simulink model "Improved_EKFSim"  (R2021b)
settings: Solver=VariableStepAuto  StartTime=0.0  StopTime=12000  RelTol=1e-3
undefined symbols (not defined in the file): sigbuilder_block
libraries: commchan3 x2
settings Model: Creator=Lenovo  LastModifiedBy=matthewathanasopoulos
settings SolverCC: AlgebraicLoopSolver=TrustRegion
settings DataIOCC: ReturnWorkspaceOutputs=off
settings DebuggingCC: SFMachineParentedDataDiag=warning  ArithmeticOperatorsInVariantConditions=warning
settings SFSimCC: SimUseLocalCustomCode=off  CustomCodeUndefinedFunction=UseInterfaceOnly
settings RTWCC: RTWUseLocalCustomCode=off

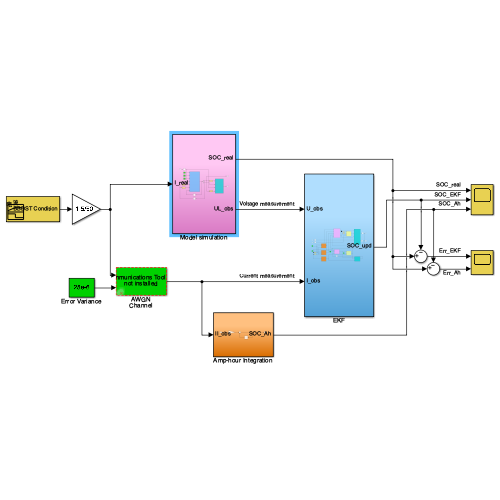
[thumbnail: Simulink's stored preview of the top-level diagram]
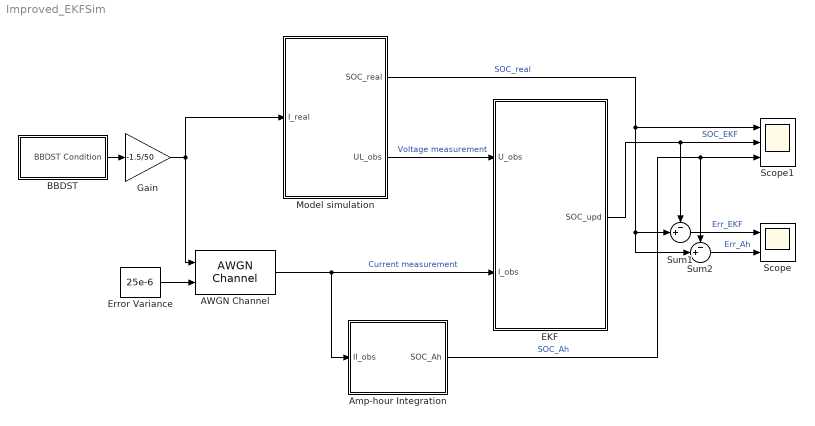
== system Improved_EKFSim ==
  AWGN Channel : commchan3/AWGN Channel  InputProcessing=Columns as channels (frame based)  seed=1  noiseMode=Variance from port  EbNodB=10  EsNodB=10  SNRdB=10  bitsPerSym=1  Ps=1  Tsym=1  variance=1
  Amp-hour Integration : Subsystem
  BBDST : Subsystem  Tag=STV Subsys  LoadFcn=sigbuilder_block('load');  StartFcn=sigbuilder_block('start');  StopFcn=sigbuilder_block('stop');  ClipboardFcn=sigbuilder_block('clipboard');  mask(Sigbuilder block){tuvar=[0:10]}
      mask help: Simulink:masks:SigbuilderBlock_MD
      mask init:
      | if ~strcmp(get_param(bdroot(gcbh),'SimulationStatus'),'stopped') tuvar = sigbuilder_block('maskInit'); end
      settings: CopyFcn=sigbuilder_block('copy');  DeleteFcn=sigbuilder_block('delete');  ModelCloseFcn=sigbuilder_block('modelClose');  PreSaveFcn=sigbuilder_block('preSave');  PauseFcn=sigbuilder_block('pause');  ContinueFcn=sigbuilder_block('continue');  NameChangeFcn=sigbuilder_block('namechange');  OpenFcn=sigbuilder_block('open',[162 96 990 471 ]);  CloseFcn=sigbuilder_block('close');
      mask Display: plot(0, 0, 100, 100,[2, 2, 32, 32, 2], [68, 8, 8, 68, 68],[32, 2], [38, 38], [32, 19, 2],[53, 60, 44], [32, 17, 17, 2],[16, 16, 31, 31]);txt = getActiveGroup(gcbh);text(2, 100, txt,'verticalAlignment', 'top');
  EKF : Subsystem
  Error Variance : Constant  Value=25e-6
  Gain : Gain  Gain=-1.5/50
  Model simulation : Subsystem
  Scope : Scope  NumInputPorts=2
  Scope1 : Scope  NumInputPorts=3
  Sum1 : Sum  Inputs=-+|
  Sum2 : Sum  Inputs=-+|
  wires:
  BBDST/1(BBDST Condition) -> Gain/1
  AWGN Channel/1 -> Amp-hour Integration/1(II_obs), EKF/2(I_obs)  "Current measurement"
  EKF/1(SOC_upd) -> Sum1/1, Scope1/2  "SOC_EKF"
  Model simulation/2(UL_obs) -> EKF/1(U_obs)  "Voltage measurement"
  Model simulation/1(SOC_real) -> Scope1/1, Sum2/2, Sum1/2  "SOC_real"
  Gain/1 -> AWGN Channel/1, Model simulation/1(I_real)
  Amp-hour Integration/1(SOC_Ah) -> Sum2/1, Scope1/3  "SOC_Ah"
  Sum1/1 -> Scope/1  "Err_EKF"
  Sum2/1 -> Scope/2  "Err_Ah"
  Error Variance/1 -> AWGN Channel/2

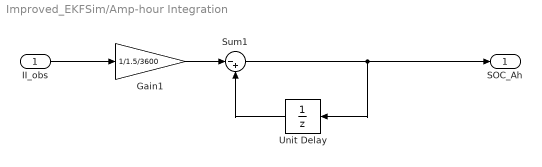
== system Improved_EKFSim/Amp-hour Integration ==
  II_obs : Inport
  Gain1 : Gain  Gain=1/1.5/3600
  Sum1 : Sum  Inputs=|-+
  Unit Delay : UnitDelay  InitialCondition=1  HasFrameUpgradeWarning=on
  SOC_Ah : Outport  VectorParamsAs1DForOutWhenUnconnected=off
  wires:
  Gain1/1 -> Sum1/1
  Sum1/1 -> SOC_Ah/1, Unit Delay/1
  II_obs/1 -> Gain1/1
  Unit Delay/1 -> Sum1/2

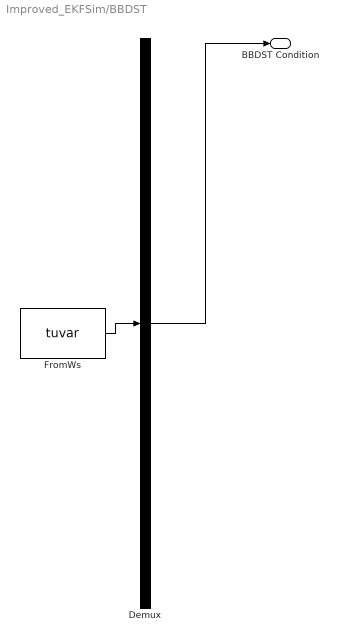
== system Improved_EKFSim/BBDST ==
  Demux : Demux  Tag=STV Demux  Outputs=1
      settings: DisplayOption=none
  FromWs : FromWorkspace  Tag=STV FromWs  VariableName=tuvar
      SigBuilderData=|
      | common.afterFinalStr = 'Extrapolate'
      | common.sampleTime = 0
      | dataSet.timeRange = [0 13328.1]
      | dataSet.name = '电流'
      | sbobj.Name = 'Signal Builder'
      | sbobj.Groups.Name = '电流'
      | sbobj.Groups.Signals.Name = 'BBDST Condition'
      | sbobj.Groups.Signals.XData = [0 0.1 0.2 0.3 0.4 0.5 0.6 0.7 0.8 0.9 1 1.1 ... (133282 elements, 1x133282)]
      | sbobj.Groups.Signals.YData = [-16.77 -16.77 -16.77 -16.77 -16.77 -16.77 -16.78 -16.79 -16.79 -16.79 -16.79 -16.79 ... (133282 elements, 1x133282)]
      | sbobj.Groups.TimeRange = [0 13328.1]
  BBDST Condition : Outport  VectorParamsAs1DForOutWhenUnconnected=off
  wires:
  Demux/1 -> BBDST Condition/1
  FromWs/1 -> Demux/1

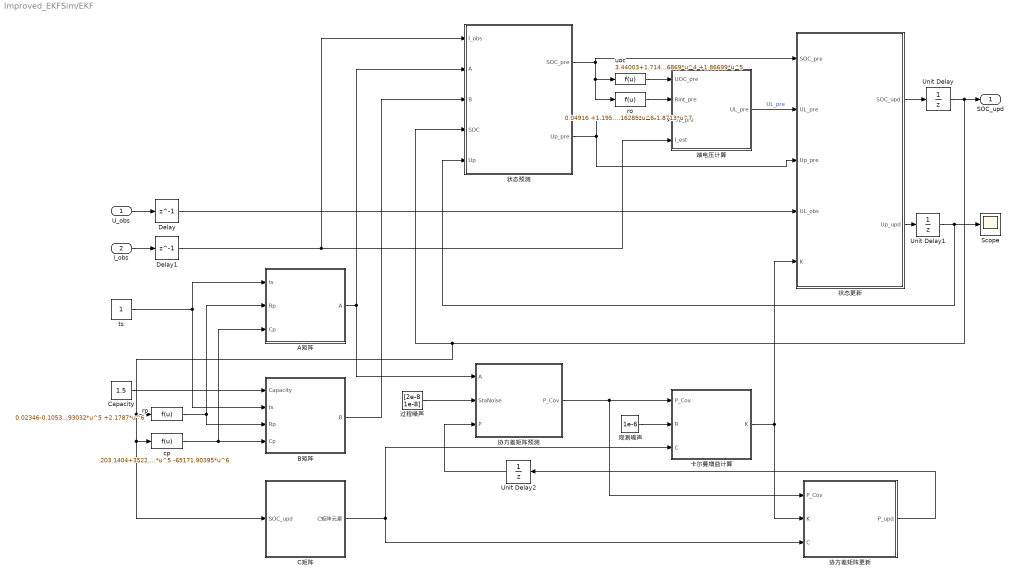
== system Improved_EKFSim/EKF ==
  U_obs : Inport
  I_obs : Inport  Port=2
  A矩阵 : Subsystem  TreatAsAtomicUnit=on
  B矩阵 : Subsystem  TreatAsAtomicUnit=on
  Capacity : Constant  Value=1.5
  C矩阵 : Subsystem  TreatAsAtomicUnit=on
  Delay : Delay  DelayLength=1  InitialCondition=0  SampleTime=1
  Delay1 : Delay  DelayLength=1  InitialCondition=0  SampleTime=1
  Scope : Scope
  Unit Delay : UnitDelay  InitialCondition=1  HasFrameUpgradeWarning=on
  Unit Delay1 : UnitDelay  HasFrameUpgradeWarning=on
  Unit Delay2 : UnitDelay  InitialCondition=[0 0 0 0]  HasFrameUpgradeWarning=on
  cp : Fcn  Expr=203.1404+3522.78847*u-31392.66753*u^2+122406.91269*u^3-227590.94382*u^4+198281.56406*u^5 -65171.90395*u^6
  ro : Fcn  Expr=0.04916 +1.19552*u-6.25333*u^2+14.24181*u^3-13.93388*u^4+2.553*u^5+4.16285*u^6-1.8713*u^7
  rp : Fcn  Expr=0.02346-0.10537*u^1+1.1371*u^2-4.55188*u^3+8.26827*u^4-6.93032*u^5 +2.1787*u^6
  ts : Constant
  uoc : Fcn  Expr=3.44003+1.71448*u -3.51247*u^2 +5.70868*u^3 -5.06869*u^4 +1.86699*u^5
  协方差矩阵更新 : MATLAB Function  TreatAsAtomicUnit=on
  协方差矩阵预测 : MATLAB Function  TreatAsAtomicUnit=on
  卡尔曼增益计算 : MATLAB Function  TreatAsAtomicUnit=on
  状态更新 : Subsystem
  状态预测 : Subsystem
  端电压计算 : Subsystem  TreatAsAtomicUnit=on
  观测噪声 : Constant  Value=1e-6
  过程噪声 : Constant  Value=[2e-8 1e-8]
  SOC_upd : Outport  VectorParamsAs1DForOutWhenUnconnected=off
  wires:
  C矩阵/1(C矩阵元素) -> 协方差矩阵更新/3(C), 卡尔曼增益计算/3(C)
  A矩阵/1(A) -> 协方差矩阵预测/1(A), 状态预测/2(A)
  rp/1 -> B矩阵/3(Rp), A矩阵/2(Rp)
  过程噪声/1 -> 协方差矩阵预测/2(StaNoise)
  cp/1 -> A矩阵/3(Cp), B矩阵/4(Cp)
  卡尔曼增益计算/1(K) -> 协方差矩阵更新/2(K), 状态更新/5(K)
  ts/1 -> B矩阵/2(ts), A矩阵/1(ts)
  ro/1 -> 端电压计算/2(Rint_pre)
  协方差矩阵更新/1(P_upd) -> Unit Delay2/1
  Capacity/1 -> B矩阵/1(Capacity)
  I_obs/1 -> Delay1/1
  观测噪声/1 -> 卡尔曼增益计算/2(R)
  U_obs/1 -> Delay/1
  uoc/1 -> 端电压计算/1(UOC_pre)
  Delay1/1 -> 端电压计算/4(I_est), 状态预测/1(I_obs)
  状态更新/2(Up_upd) -> Unit Delay1/1
  状态更新/1(SOC_upd) -> Unit Delay/1
  端电压计算/1(UL_pre) -> 状态更新/2(UL_pre)  "UL_pre"
  Delay/1 -> 状态更新/4(UL_obs)
  状态预测/1(SOC_pre) -> 状态更新/1(SOC_pre), ro/1, uoc/1
  状态预测/2(Up_pre) -> 状态更新/3(Up_pre), 端电压计算/3(Up_pre)
  Unit Delay/1 -> 状态预测/4(SOC), C矩阵/1(SOC_upd), cp/1, rp/1, SOC_upd/1
  Unit Delay1/1 -> 状态预测/5(Up), Scope/1
  B矩阵/1(B) -> 状态预测/3(B)
  协方差矩阵预测/1(P_Cov) -> 协方差矩阵更新/1(P_Cov), 卡尔曼增益计算/1(P_Cov)
  Unit Delay2/1 -> 协方差矩阵预测/3(P)

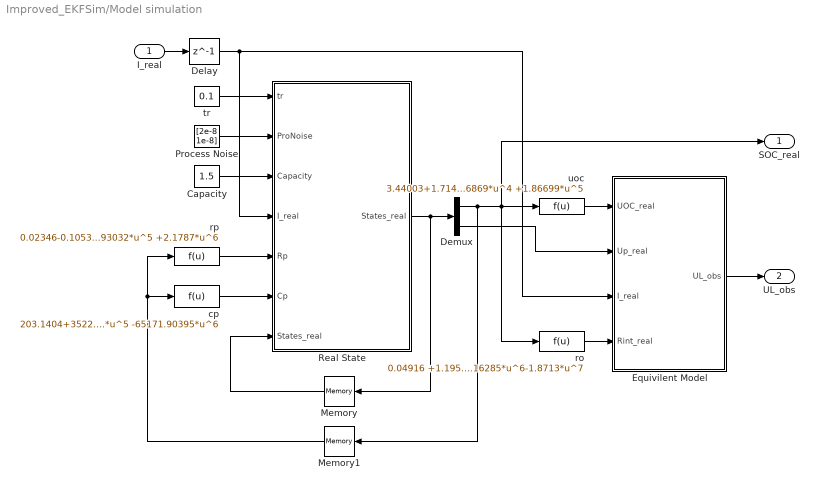
== system Improved_EKFSim/Model simulation ==
  I_real : Inport
  Capacity : Constant  Value=1.5
  Delay : Delay  DelayLength=1  InitialCondition=0  SampleTime=0.1
  Demux : Demux  Outputs=2
  Equivilent Model : Subsystem  TreatAsAtomicUnit=on
  Memory : Memory  InitialCondition=[1;0]
  Memory1 : Memory  InitialCondition=1
  Process Noise : Constant  Value=[2e-8 1e-8]
  Real State : MATLAB Function  TreatAsAtomicUnit=on
  cp : Fcn  Expr=203.1404+3522.78847*u-31392.66753*u^2+122406.91269*u^3-227590.94382*u^4+198281.56406*u^5 -65171.90395*u^6
  ro : Fcn  Expr=0.04916 +1.19552*u-6.25333*u^2+14.24181*u^3-13.93388*u^4+2.553*u^5+4.16285*u^6-1.8713*u^7
  rp : Fcn  Expr=0.02346-0.10537*u^1+1.1371*u^2-4.55188*u^3+8.26827*u^4-6.93032*u^5 +2.1787*u^6
  tr : Constant  Value=0.1
  uoc : Fcn  Expr=3.44003+1.71448*u -3.51247*u^2 +5.70868*u^3 -5.06869*u^4 +1.86699*u^5
  SOC_real : Outport  VectorParamsAs1DForOutWhenUnconnected=off
  UL_obs : Outport  Port=2  VectorParamsAs1DForOutWhenUnconnected=off
  wires:
  Demux/2 -> Equivilent Model/2(Up_real)
  rp/1 -> Real State/5(Rp)
  tr/1 -> Real State/1(tr)
  Real State/1(States_real) -> Demux/1, Memory/1
  Memory1/1 -> rp/1, cp/1
  ro/1 -> Equivilent Model/4(Rint_real)
  cp/1 -> Real State/6(Cp)
  Capacity/1 -> Real State/3(Capacity)
  uoc/1 -> Equivilent Model/1(UOC_real)
  Memory/1 -> Real State/7("States_real ")
  Process Noise/1 -> Real State/2(ProNoise)
  Equivilent Model/1(UL_obs) -> UL_obs/1
  Delay/1 -> Real State/4(I_real), Equivilent Model/3(I_real)
  Demux/1 -> uoc/1, SOC_real/1, ro/1, Memory1/1
  I_real/1 -> Delay/1

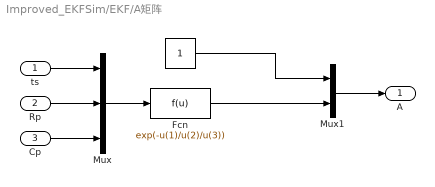
== system Improved_EKFSim/EKF/A矩阵 ==
  ts : Inport
  Rp : Inport  Port=2
  Cp : Inport  Port=3
  " " : Constant
  Fcn : Fcn  Expr=exp(-u(1)/u(2)/u(3))
  Mux : Mux  Inputs=3
  Mux1 : Mux  Inputs=2
  A : Outport  VectorParamsAs1DForOutWhenUnconnected=off
  wires:
  Rp/1 -> Mux/2
  Fcn/1 -> Mux1/2
  ts/1 -> Mux/1
  Cp/1 -> Mux/3
  Mux/1 -> Fcn/1
  " "/1 -> Mux1/1
  Mux1/1 -> A/1

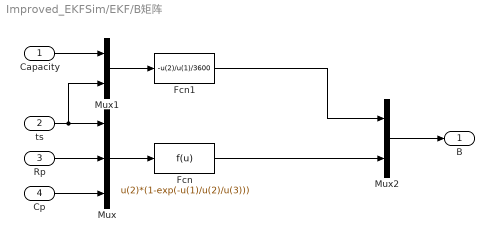
== system Improved_EKFSim/EKF/B矩阵 ==
  Capacity : Inport
  ts : Inport  Port=2
  Rp : Inport  Port=3
  Cp : Inport  Port=4
  Fcn : Fcn  Expr=u(2)*(1-exp(-u(1)/u(2)/u(3)))
  Fcn1 : Fcn  Expr=-u(2)/u(1)/3600
  Mux : Mux  Inputs=3
  Mux1 : Mux  Inputs=2
  Mux2 : Mux  Inputs=2
  B : Outport  VectorParamsAs1DForOutWhenUnconnected=off
  wires:
  Rp/1 -> Mux/2
  ts/1 -> Mux1/2, Mux/1
  Cp/1 -> Mux/3
  Mux/1 -> Fcn/1
  Capacity/1 -> Mux1/1
  Mux1/1 -> Fcn1/1
  Fcn/1 -> Mux2/2
  Fcn1/1 -> Mux2/1
  Mux2/1 -> B/1

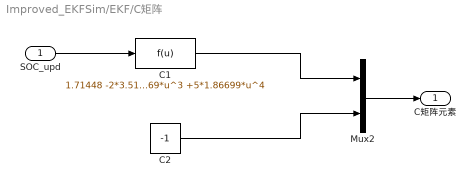
== system Improved_EKFSim/EKF/C矩阵 ==
  SOC_upd : Inport
  C1 : Fcn  Expr=1.71448 -2*3.51247*u +3*5.70868*u^2 -4*5.06869*u^3 +5*1.86699*u^4
  C2 : Constant  Value=-1
  Mux2 : Mux  Inputs=2
  C矩阵元素 : Outport  VectorParamsAs1DForOutWhenUnconnected=off
  wires:
  C1/1 -> Mux2/1
  C2/1 -> Mux2/2
  Mux2/1 -> C矩阵元素/1
  SOC_upd/1 -> C1/1

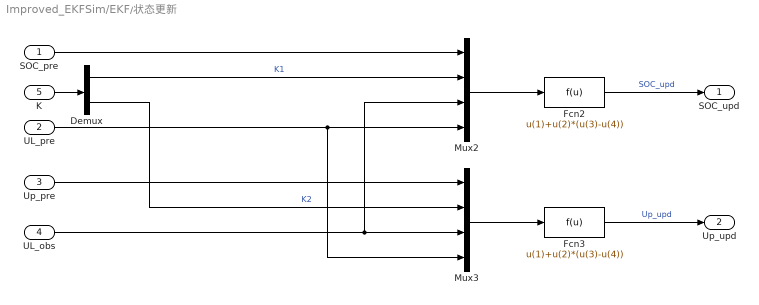
== system Improved_EKFSim/EKF/状态更新 ==
  SOC_pre : Inport
  UL_pre : Inport  Port=2
  Up_pre : Inport  Port=3
  UL_obs : Inport  Port=4
  K : Inport  Port=5
  Demux : Demux  Outputs=2
  Fcn2 : Fcn  Expr=u(1)+u(2)*(u(3)-u(4))
  Fcn3 : Fcn  Expr=u(1)+u(2)*(u(3)-u(4))
  Mux2 : Mux
  Mux3 : Mux
  SOC_upd : Outport  VectorParamsAs1DForOutWhenUnconnected=off
  Up_upd : Outport  Port=2  VectorParamsAs1DForOutWhenUnconnected=off
  wires:
  Fcn3/1 -> Up_upd/1  "Up_upd"
  Demux/1 -> Mux2/2  "K1"
  Demux/2 -> Mux3/2  "K2"
  Mux2/1 -> Fcn2/1
  Mux3/1 -> Fcn3/1
  K/1 -> Demux/1
  UL_obs/1 -> Mux3/3, Mux2/3
  UL_pre/1 -> Mux3/4, Mux2/4
  Up_pre/1 -> Mux3/1
  SOC_pre/1 -> Mux2/1
  Fcn2/1 -> SOC_upd/1  "SOC_upd"

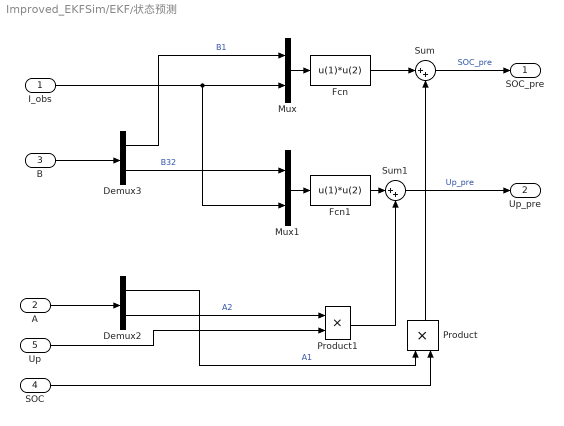
== system Improved_EKFSim/EKF/状态预测 ==
  I_obs : Inport
  A : Inport  Port=2
  B : Inport  Port=3
  SOC : Inport  Port=4
  Up : Inport  Port=5
  Demux2 : Demux  Outputs=2
  Demux3 : Demux  Outputs=2
  Fcn : Fcn  Expr=u(1)*u(2)
  Fcn1 : Fcn  Expr=u(1)*u(2)
  Mux : Mux  Inputs=2
  Mux1 : Mux  Inputs=2
  Product : Product
  Product1 : Product
  Sum : Sum  Inputs=|++
  Sum1 : Sum  Inputs=|++
  SOC_pre : Outport  VectorParamsAs1DForOutWhenUnconnected=off
  Up_pre : Outport  Port=2  VectorParamsAs1DForOutWhenUnconnected=off
  wires:
  Fcn/1 -> Sum/1
  Demux2/2 -> Product1/1  "A2"
  A/1 -> Demux2/1
  Demux3/1 -> Mux/1  "B1"
  Demux2/1 -> Product/1  "A1"
  SOC/1 -> Product/2
  Fcn1/1 -> Sum1/1
  Mux/1 -> Fcn/1
  Mux1/1 -> Fcn1/1
  Product/1 -> Sum/2
  Demux3/2 -> Mux1/1  "B32"
  Sum1/1 -> Up_pre/1  "Up_pre"
  I_obs/1 -> Mux1/2, Mux/2
  Up/1 -> Product1/2
  Product1/1 -> Sum1/2
  Sum/1 -> SOC_pre/1  "SOC_pre"
  B/1 -> Demux3/1

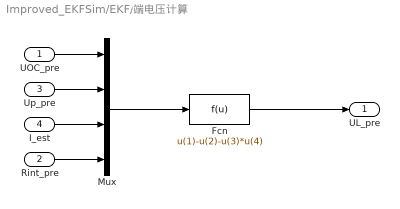
== system Improved_EKFSim/EKF/端电压计算 ==
  UOC_pre : Inport
  Rint_pre : Inport  Port=2
  Up_pre : Inport  Port=3
  I_est : Inport  Port=4
  Fcn : Fcn  Expr=u(1)-u(2)-u(3)*u(4)
  Mux : Mux
  UL_pre : Outport  VectorParamsAs1DForOutWhenUnconnected=off
  wires:
  I_est/1 -> Mux/3
  Up_pre/1 -> Mux/2
  Rint_pre/1 -> Mux/4
  Mux/1 -> Fcn/1
  Fcn/1 -> UL_pre/1
  UOC_pre/1 -> Mux/1

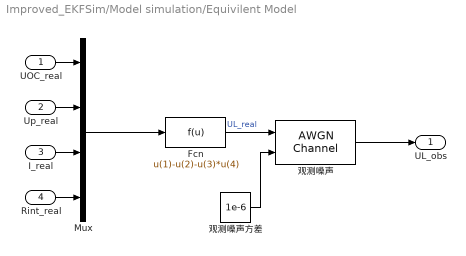
== system Improved_EKFSim/Model simulation/Equivilent Model ==
  UOC_real : Inport
  Up_real : Inport  Port=2
  I_real : Inport  Port=3
  Rint_real : Inport  Port=4
  Fcn : Fcn  Expr=u(1)-u(2)-u(3)*u(4)
  Mux : Mux
  观测噪声 : commchan3/AWGN Channel  InputProcessing=Columns as channels (frame based)  seed=1  noiseMode=Variance from port  EbNodB=10  EsNodB=10  SNRdB=10  bitsPerSym=1  Ps=1  Tsym=1  variance=1
  观测噪声方差 : Constant  Value=1e-6
  UL_obs : Outport  VectorParamsAs1DForOutWhenUnconnected=off
  wires:
  Fcn/1 -> 观测噪声/1  "UL_real"
  Mux/1 -> Fcn/1
  UOC_real/1 -> Mux/1
  Up_real/1 -> Mux/2
  I_real/1 -> Mux/3
  Rint_real/1 -> Mux/4
  观测噪声/1 -> UL_obs/1
  观测噪声方差/1 -> 观测噪声/2

== matlab function Improved_EKFSim/Model simulation/Real State ==
  data: tr input; States_real output; ProNoise input; Capacity input; I_real input; Rp input; Cp input; States_real input
function States_real = StatReal(tr, ProNoise, Capacity, I_real, Rp, Cp, States_real)
    tao = Rp * Cp;
    Qs = ProNoise(1);
    Qu = ProNoise(2);
    
    A2=exp(-tr/tao);
    A=[1 0;0 A2];  % State transformation matrix
    B1 = -tr/(Capacity*3600);
    B2=Rp*(1-exp(-tr/tao));  
    B=[B1;B2];  % Input control matrix
    States_real = A*States_real + B*I_real + [sqrt(Qs)*randn;sqrt(Qu)*randn];  % 实际过程模拟以 0.1s 更新一次

== matlab function Improved_EKFSim/EKF/协方差矩阵预测 ==
  data: A input; P_Cov output; StaNoise input; P input
function P_Cov = CovMat(A, StaNoise, P)
A1 = [A(1) 0;0 A(2)];
Qs = StaNoise(1);
Qu = StaNoise(2);
P1 = [P(1) P(2) ; P(3) P(4)];
P2 = A1*P1*A1' + [Qs 0;0 Qu];  % 协方差矩阵预测
P_Cov = [P2(1,1) P2(1,2) P2(2,1) P2(2,2)];

== matlab function Improved_EKFSim/EKF/卡尔曼增益计算 ==
  data: P_Cov input; R input; C input; K output
function K = KalmanGain(P_Cov, R, C)
C1 = [C(1) C(2)];
P = [P_Cov(1) P_Cov(2) ;  P_Cov(3) P_Cov(4)];
K = P*C1'* (C1*P*C1'+R)^(-1);  % 增益

== matlab function Improved_EKFSim/EKF/协方差矩阵更新 ==
  data: P_Cov input; K input; C input; P_upd output
function P_upd = CovUpd(P_Cov, K, C)
C = [C(1) C(2)];
P = [P_Cov(1) P_Cov(2) ; P_Cov(3) P_Cov(4)];
P1 = P - K * C * P;  % 协方差矩阵更新
P_upd = [P1(1,1) P1(1,2) P1(2,1) P1(2,2)];
